simulink library "xpcaddidatalib"  (Simulink 6.0)
settings: Solver=ode45  SolverMode=SingleTasking  StartTime=0.0  StopTime=10.0  RelTol=1e-3
undefined symbols (not defined in the file or in its folder): mapci1710
settings Model: Creator=adowd  LastModifiedBy=adowd
settings DataIOCC: SignalLoggingName=logsOut
settings OptimizationCC: BooleanDataType=off
settings DebuggingCC: CheckExecutionContextPreStartOutputMsg=on  CheckExecutionContextRuntimeOutputMsg=on  SolverPrmCheckMsg=none
settings HardwareCC: TargetUnknown=on
settings GRTTargetCC: UtilityFuncGeneration=Automatic  LifeSpan=inf
settings SFSimCC: SFSimApplyToAllLibs=on  SFSimBuildMode=Incremental

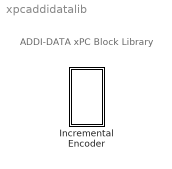
== system xpcaddidatalib ==
  note: ADDI-DATA xPC Block Library
  Incremental Encoder : Subsystem  EnableExecutionContextPropagation=on

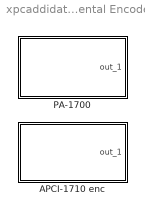
== system xpcaddidatalib/Incremental Encoder ==
  "APCI-1710 enc " : Subsystem  InitFcn=mapci1710(1);  EnableExecutionContextPropagation=on  mask(Incremental Encoder Module){module=1, reset=Virtual Absolute, mode=single, hyst=off, res=4096, sampletime=0.001, pci_dev=-1}
      mask prompts: module "Function module:"; reset "Type of evaluation:"; hyst "Hysteresis:"; res "Resolution:"; sampletime "Sample time:"; pci_dev "PCI slot (-1: autosearch):"
      mask help:
      | ADDI-DATA
      | APCI-1710
      | Incremental Encoder
      mask Help: helpview(fullfile(docroot, 'mapfiles', 'xpc.map'), 'ADDI-DATA_APCI-1710-enc_Encoder')
      mask StyleString: popup(1|2|3|4),popup(Virtual Absolute|Reset and Index Output Up-Dating),popup(single|double|quadruple),popup(off|on),edit,edit,edit
      mask Display: disp('APCI-1710\nADDI-DATA\nIncremental Encoder')
  "PA-1700 " : Subsystem  EnableExecutionContextPropagation=on  mask(Incremental Encoder Module){counter=1, mode=single, hyst=off, res=4096, sampletime=0.001, baseaddress=0x300}
      mask prompts: hyst "Hysteresis:"; res "Resolution:"; sampletime "Sample time:"; baseaddress "Base address (i.e. 0xd000):"
      mask help:
      | ADDI-DATA
      | PA-1700
      | Incremental Encoder
      mask init:
      | reset=1;
      | baseaddress=hex2dec(baseaddress(3:end));
      mask Help: helpview(fullfile(docroot, 'mapfiles', 'xpc.map'), 'ADDI-DATA_PA-1700_Encoder')
      mask StyleString: popup(1|2|3),popup(single|double|quadruple),popup(off|on),edit,edit,edit
      mask Display: disp('PA1700\nADDI-DATA\nIncremental Encoder')

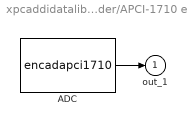
== system xpcaddidatalib/Incremental Encoder/APCI-1710 enc  ==
  ADC : S-Function  FunctionName=encadapci1710  Parameters=reset,module, mode, hyst, res, sampletime, pci_dev
  out_1 : Outport  InitialOutput=0
  wires:
  ADC/1 -> out_1/1

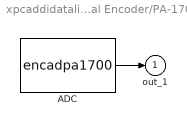
== system xpcaddidatalib/Incremental Encoder/PA-1700  ==
  ADC : S-Function  FunctionName=encadpa1700  Parameters=reset,counter, mode, hyst, res, sampletime, baseaddress
  out_1 : Outport  InitialOutput=0
  wires:
  ADC/1 -> out_1/1
